simulink model "plant_model"  (R2023b)
settings: Solver=VariableStepAuto  StartTime=0.0  StopTime=Tfin  RelTol=1e-3
values from neighbouring files (symbols this model uses):
  x0 = [r0;v0; tot_mass]    [es2.m]    (also in nmpc_design_template.m = [r0; v0; totmass])
undefined symbols (not defined in the file or in its folder): spacecraft_dynamics
settings Model: Creator=s331564  LastModifiedBy=luigi

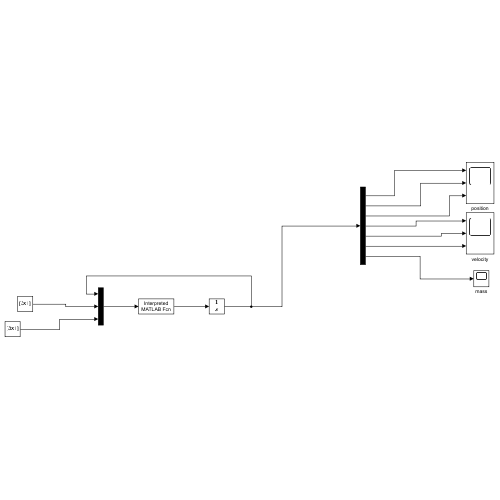
[thumbnail: Simulink's stored preview of the top-level diagram]
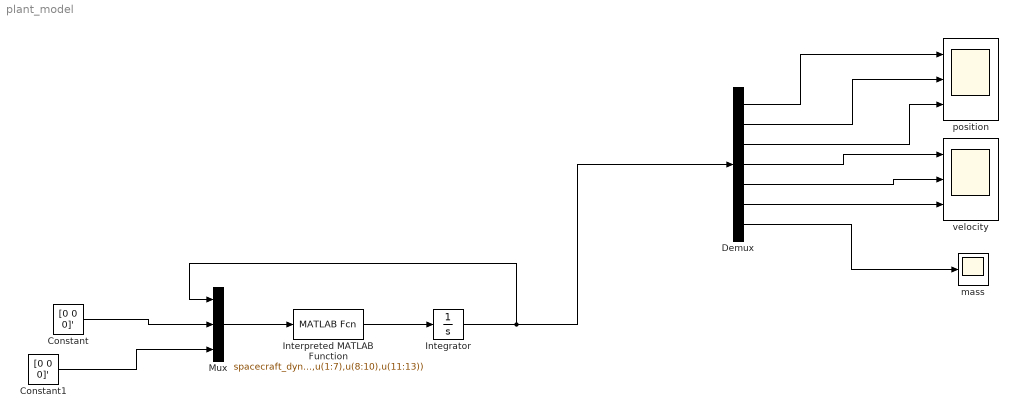
== system plant_model ==
  Constant : Constant  Value=[0 0 0]'
  Constant1 : Constant  Value=[0 0 0]'
  Demux : Demux  Outputs=7
  Integrator : Integrator  InitialCondition=x0
  Interpreted MATLAB Function : MATLABFcn  MATLABFcn=spacecraft_dynamics(0,u(1:7),u(8:10),u(11:13))
  Mux : Mux  Inputs=3
  mass : Scope
  position : Scope  NumInputPorts=3
  velocity : Scope  NumInputPorts=3
  wires:
  Demux/2 -> position/2
  Demux/6 -> velocity/3
  Interpreted MATLAB Function/1 -> Integrator/1
  Demux/3 -> position/3
  Demux/4 -> velocity/1
  Demux/1 -> position/1
  Mux/1 -> Interpreted MATLAB Function/1
  Demux/7 -> mass/1
  Integrator/1 -> Demux/1, Mux/1
  Demux/5 -> velocity/2
  Constant/1 -> Mux/2
  Constant1/1 -> Mux/3
